simulink model "droneSim"  (R2020a)
settings: Solver=VariableStepAuto  StartTime=0.0  StopTime=10  RelTol=1e-3
model workspace (MAT data in the model file):
  b = 0.000146
  dragCoef = 1
  k = 0.026
  l = 0.17
  mass = 1.104
libraries: shared6dof x1, simulink_extras x1
settings Model: Creator=rpogl  LastModifiedBy=rpogl

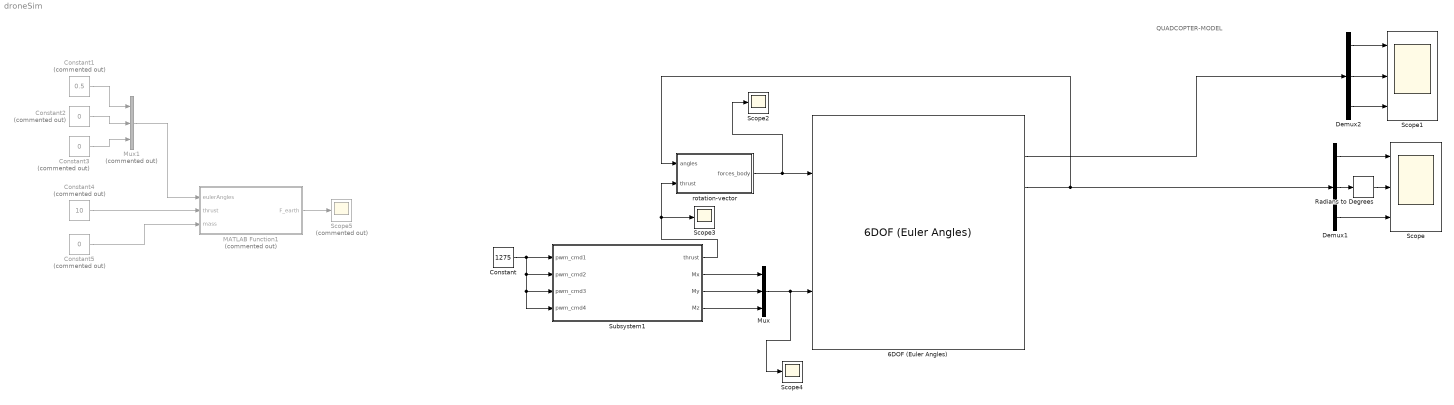
== system droneSim ==
  note: QUADCOPTER-MODEL
  6DOF (Euler Angles) : shared6dof/6DOF (Euler Angles)  units=Metric (MKS)  mtype=Fixed  rep=Euler Angles  xme_0=[0 0 0]  Vm_0=[0 0 0]  eul_0=[0 0 0]  pm_0=[0 0 0]  mass_0=mass  mass_e=0.5  mass_f=2.0  inertia=[0.0063 0 0; 0 0.0063 0;0 0 0.21425]  inertia_e=eye(3)  inertia_f=2*eye(3)  k_quat=1.0  vre_flag=on  abi_flag=off  aMode=0  xme_statename=''  Vm_statename=''  eul_statename=''  quat_statename=''  pm_statename=''  mass_statename=''
      settings: SourceProductBaseCode=AE,PW,MT,VE,VP
  Constant : Constant  Value=1275
  Constant1 : Constant  Commented=on  Value=0.5
  Constant2 : Constant  Commented=on  Value=0
  Constant3 : Constant  Commented=on  Value=0
  Constant4 : Constant  Commented=on  Value=10
  Constant5 : Constant  Commented=on  Value=0
  Demux1 : Demux  Outputs=3
  Demux2 : Demux  Outputs=3
  MATLAB Function1 : MATLAB Function  Commented=on  TreatAsAtomicUnit=on
  Mux : Mux  Inputs=3
  Mux1 : Mux  Commented=on  Inputs=3
  Radians to Degrees : simulink_extras/Transformations/Radians to Degrees
  Scope : Scope  NumInputPorts=3
  Scope1 : Scope  NumInputPorts=3
  Scope2 : Scope
  Scope3 : Scope
  Scope4 : Scope
  Scope5 : Scope  Commented=on
  Subsystem1 : Subsystem
  rotation-vector : Subsystem
  wires:
  Demux1/1 -> Scope/1
  Demux1/2 -> Radians to Degrees/1
  Demux1/3 -> Scope/3
  6DOF (Euler Angles)/2 -> Demux2/1
  Demux2/1 -> Scope1/1
  Demux2/2 -> Scope1/2
  Demux2/3 -> Scope1/3
  Radians to Degrees/1 -> Scope/2
  Subsystem1/2(Mx) -> Mux/1
  Subsystem1/3(My) -> Mux/2
  Subsystem1/4(Mz) -> Mux/3
  Mux/1 -> Scope4/1, 6DOF (Euler Angles)/2
  MATLAB Function1/1(F_earth) -> Scope5/1
  Mux1/1 -> MATLAB Function1/1(eulerAngles)
  Constant3/1 -> Mux1/3
  Constant2/1 -> Mux1/2
  Constant1/1 -> Mux1/1
  Constant5/1 -> MATLAB Function1/3(mass)
  Constant4/1 -> MATLAB Function1/2(thrust)
  rotation-vector/1(forces_body) -> Scope2/1, 6DOF (Euler Angles)/1
  6DOF (Euler Angles)/3 -> rotation-vector/1(angles), Demux1/1
  Subsystem1/1(thrust) -> rotation-vector/2(thrust), Scope3/1
  Constant/1 -> Subsystem1/4(pwm_cmd4), Subsystem1/3(pwm_cmd3), Subsystem1/2(pwm_cmd2), Subsystem1/1(pwm_cmd1)

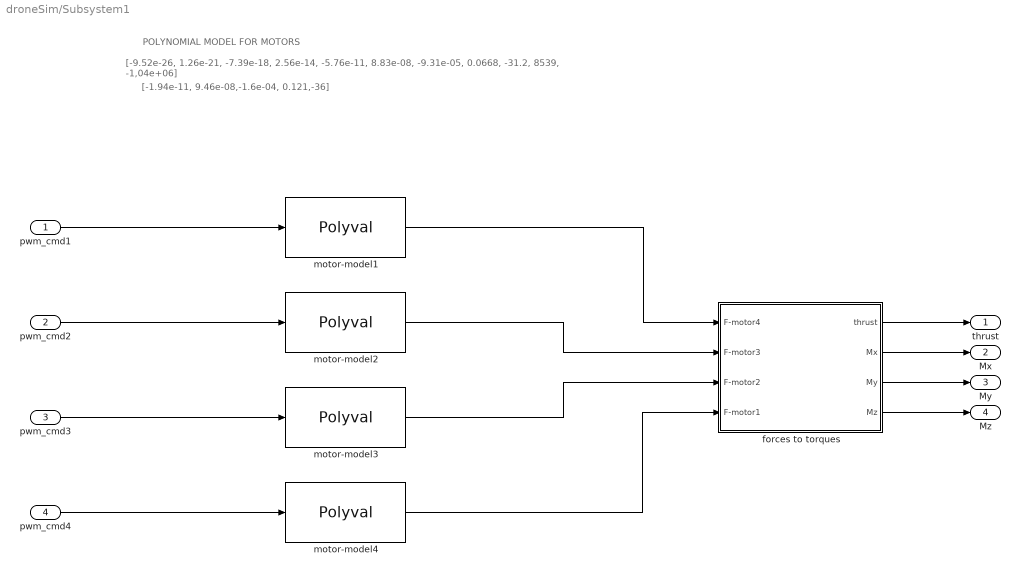
== system droneSim/Subsystem1 ==
  note: POLYNOMIAL MODEL FOR MOTORS
  note: [-9.52e-26, 1.26e-21, -7.39e-18, 2.56e-14, -5.76e-11, 8.83e-08, -9.31e-05, 0.0668, -31.2, 8539, -1,04e+06]
  note: [-1.94e-11, 9.46e-08,-1.6e-04, 0.121,-36]
  pwm_cmd1 : Inport
  pwm_cmd2 : Inport  Port=2
  pwm_cmd3 : Inport  Port=3
  pwm_cmd4 : Inport  Port=4
  forces to torques : Subsystem
  motor-model{1..4} (4 alike) : Polyval  Coefs=[-1.94e-11, 9.46e-08,-1.6e-04, 0.121,-36]
  thrust : Outport
  Mx : Outport  Port=2
  My : Outport  Port=3
  Mz : Outport  Port=4
  wires:
  forces to torques/2(Mx) -> Mx/1
  forces to torques/1(thrust) -> thrust/1
  forces to torques/3(My) -> My/1
  forces to torques/4(Mz) -> Mz/1
  pwm_cmd2/1 -> motor-model2/1
  pwm_cmd1/1 -> motor-model1/1
  pwm_cmd3/1 -> motor-model3/1
  pwm_cmd4/1 -> motor-model4/1
  motor-model1/1 -> forces to torques/1(F-motor4)
  motor-model2/1 -> forces to torques/2(F-motor3)
  motor-model3/1 -> forces to torques/3(F-motor2)
  motor-model4/1 -> forces to torques/4(F-motor1)

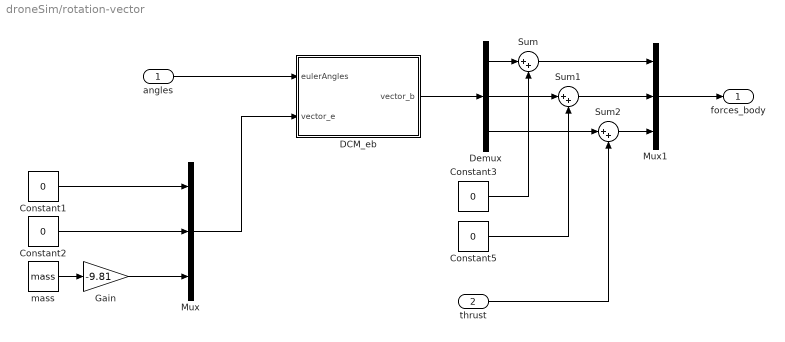
== system droneSim/rotation-vector ==
  angles : Inport
  thrust : Inport  Port=2
  Constant{1..3,5} (4 alike) : Constant  Value=0
  DCM_eb : MATLAB Function  TreatAsAtomicUnit=on
  Demux : Demux  Outputs=3
  Gain : Gain  Gain=-9.81
  Mux : Mux  Inputs=3
  Mux1 : Mux  Inputs=3
  Sum : Sum  Inputs=|++
  Sum1 : Sum  Inputs=|++
  Sum2 : Sum  Inputs=|++
  mass : Constant  Value=mass
  forces_body : Outport
  wires:
  mass/1 -> Gain/1
  Constant2/1 -> Mux/2
  Gain/1 -> Mux/3
  Constant1/1 -> Mux/1
  Mux/1 -> DCM_eb/2(vector_e)
  Mux1/1 -> forces_body/1
  Demux/1 -> Sum/1
  Sum/1 -> Mux1/1
  Demux/3 -> Sum2/1
  Sum2/1 -> Mux1/3
  Demux/2 -> Sum1/1
  Sum1/1 -> Mux1/2
  Constant3/1 -> Sum/2
  Constant5/1 -> Sum1/2
  thrust/1 -> Sum2/2
  DCM_eb/1(vector_b) -> Demux/1
  angles/1 -> DCM_eb/1(eulerAngles)

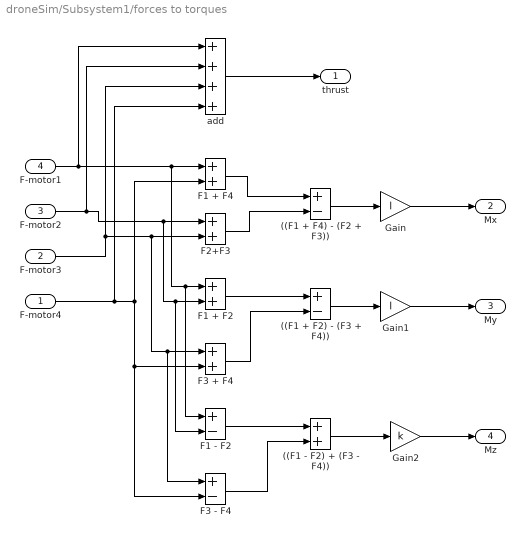
== system droneSim/Subsystem1/forces to torques ==
  F-motor4 : Inport
  F-motor3 : Inport  Port=2
  F-motor2 : Inport  Port=3
  F-motor1 : Inport  Port=4
  ((F1 + F2) - (F3 + F4)) : Sum  Inputs=+-
  ((F1 + F4) - (F2 + F3)) : Sum  Inputs=+-
  ((F1 - F2) + (F3 - F4)) : Sum
  F1 + F2 : Sum
  F1 + F4 : Sum
  F1 - F2 : Sum  Inputs=+-
  F2+F3 : Sum
  F3 + F4 : Sum
  F3 - F4 : Sum  Inputs=+-
  Gain : Gain  Gain=l
  Gain1 : Gain  Gain=l
  Gain2 : Gain  Gain=k
  add : Sum  Inputs=++++
  thrust : Outport
  Mx : Outport  Port=2
  My : Outport  Port=3
  Mz : Outport  Port=4
  wires:
  Gain1/1 -> My/1
  F1 + F4/1 -> ((F1 + F4) - (F2 + F3))/1
  F-motor1/1 -> add/1, F1 - F2/1, F1 + F2/1, F1 + F4/1
  F-motor4/1 -> add/4, F3 - F4/2, F3 + F4/2, F1 + F4/2
  F2+F3/1 -> ((F1 + F4) - (F2 + F3))/2
  ((F1 + F2) - (F3 + F4))/1 -> Gain1/1
  add/1 -> thrust/1
  F-motor3/1 -> add/3, F3 - F4/1, F3 + F4/1, F2+F3/2
  F-motor2/1 -> add/2, F1 - F2/2, F1 + F2/2, F2+F3/1
  F3 + F4/1 -> ((F1 + F2) - (F3 + F4))/2
  F1 + F2/1 -> ((F1 + F2) - (F3 + F4))/1
  F3 - F4/1 -> ((F1 - F2) + (F3 - F4))/2
  Gain/1 -> Mx/1
  ((F1 + F4) - (F2 + F3))/1 -> Gain/1
  F1 - F2/1 -> ((F1 - F2) + (F3 - F4))/1
  ((F1 - F2) + (F3 - F4))/1 -> Gain2/1
  Gain2/1 -> Mz/1

== matlab function droneSim/rotation-vector/DCM_eb ==
  data: eulerAngles input; vector_b output; vector_e input
function vector_b = fcn(eulerAngles, vector_e)
phi = eulerAngles(1);
theta = eulerAngles(2);
psi = eulerAngles(3);

R_x = [1 0 0;
       0 cos(phi) sin(phi);
       0 -sin(phi) cos(phi)];

% Matrice di rotazione per l'asse y (pitch)
R_y = [cos(theta) 0 -sin(theta);
       0 1 0;
       sin(theta) 0 cos(theta)];

% Matrice di rotazione per l'asse z (yaw)
R_z = [cos(psi) sin(psi) 0;
       -sin(psi) cos(psi) 0;
       0 0 1];

% Matrice di rotazione da Earth a Body
R_eb = R_z * R_y * R_x;

vector_b =R_eb * vector_e;

== matlab function droneSim/MATLAB Function1 ==
  data: eulerAngles input; F_earth output; thrust input; mass input
function F_earth = fcn(eulerAngles , thrust , mass)

phi = eulerAngles(1);
theta = eulerAngles(2);
psi = eulerAngles(3);

Rx = [1 0 0; 0 cos(phi) -sin(phi); 0 sin(phi) cos(phi)];
Ry = [cos(theta) 0 sin(theta); 0 1 0; -sin(theta) 0 cos(theta)];
Rz = [cos(psi) -sin(psi) 0; sin(psi) cos(psi) 0; 0 0 1];

R = Rx * Ry * Rz;

FORCES = mass * [0 0 -9.81]' + R*[0 0 thrust]';
F_earth = FORCES;
